simulink model "motor_position_controlR20011a"  (Simulink 7.7)
settings: Solver=ode45  StartTime=0.0  StopTime=10.0  RelTol=1e-3
settings Model: Creator=arturogilaparicio  LastModifiedBy=arturogilaparicio
settings DataIOCC: SignalLoggingSaveFormat=Dataset
settings OptimizationCC: ExpressionDepthLimit=128
settings DebuggingCC: UnderspecifiedInitializationDetection=Simplified  MergeDetectMultiDrivingBlocksExec=error  SolverPrmCheckMsg=none  FcnCallInpInsideContextMsg=Enable All  StateNameClashWarn=none
settings CodeAppCC: CustomSymbolStrType=$N$R$M_T
settings GRTTargetCC: TargetFunctionLibrary=C89/C90 (ANSI)

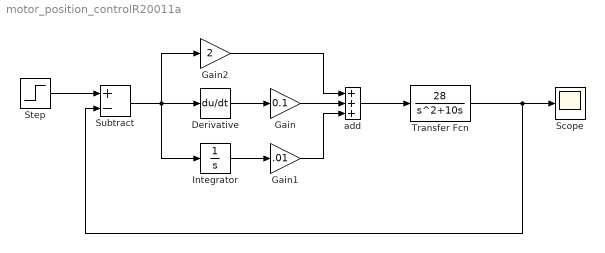
== system motor_position_controlR20011a ==
  Derivative : Derivative
  Gain : Gain  Gain=0.1
  Gain1 : Gain  Gain=.01
  Gain2 : Gain  Gain=2
  Integrator : Integrator
  Scope : Scope
  Step : Step  Time=0  After=5  SampleTime=0
  Subtract : Sum  Inputs=+-
  Transfer Fcn : TransferFcn  Numerator=[28]  Denominator=[1 10 0]
  add : Sum  Inputs=+++
  wires:
  add/1 -> Transfer Fcn/1
  Gain/1 -> add/2
  Gain2/1 -> add/1
  Gain1/1 -> add/3
  Derivative/1 -> Gain/1
  Integrator/1 -> Gain1/1
  Subtract/1 -> Integrator/1, Gain2/1, Derivative/1
  Step/1 -> Subtract/1
  Transfer Fcn/1 -> Scope/1, Subtract/2
